simulink model "VTOL_CONTROL_closedloop"  (R2025b)
settings: Solver=VariableStepAuto  StartTime=0.0  StopTime=100  RelTol=1e-3
model workspace (MAT data in the model file):
  M = 1
undefined symbols (not defined in the file): magnitude
libraries: slpidlib x2
settings Model: Creator=Admin  LastModifiedBy=Admin

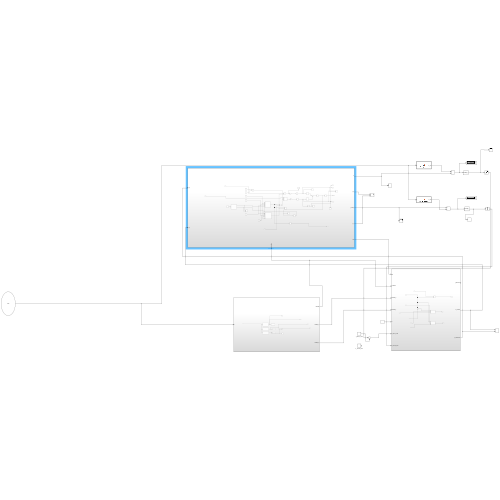
[thumbnail: Simulink's stored preview of the top-level diagram]
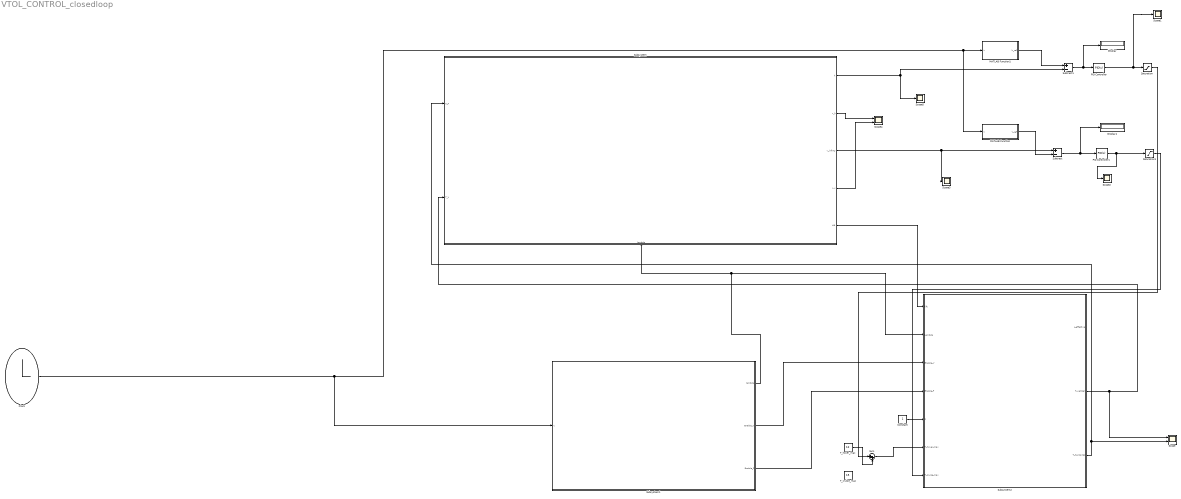
== system VTOL_CONTROL_closedloop ==
  Clock : Clock
      settings: Decimation=100
  Constant : Constant
  Display : Display
  Display1 : Display
  MATLAB Function : MATLAB Function  TreatAsAtomicUnit=on
  MATLAB Function1 : MATLAB Function  TreatAsAtomicUnit=on
  PID Controller : slpidlib/PID Controller  Controller=PID  Form=Parallel  TimeDomain=Continuous-time  UseExternalTs=off  SampleTime=-1  IntegratorMethod=Forward Euler  FilterMethod=Forward Euler  ControllerParametersSource=internal  P=40  I=0  UseKiTs=off  D=25  UseExternalDerivativeSource=off  N=100  UseFilter=on  TunerSelectOption=Transfer Function Based (PID Tuner App)  InitialConditionSource=internal  InitialConditionForIntegrator=0  InitialConditionForFilter=0  DifferentiatorICPrevScaledInput=0  ExternalReset=none  TrackingMode=off  Kt=1  LimitOutput=off  SatLimitsSource=internal  UpperSaturationLimit=inf  LowerSaturationLimit=-inf  LinearizeAsGain=on  AntiWindupMode=none  Kb=1  LimitIntegrator=off  UpperIntegratorSaturationLimit=inf  LowerIntegratorSaturationLimit=-inf  POutMin=[]  POutMax=[]  IOutMin=[]  IOutMax=[]  DOutMin=[]  DOutMax=[]  NOutMin=[]  NOutMax=[]  SumOutMin=[]  SumOutMax=[]  SaturationOutMin=[]  SaturationOutMax=[]  PParamMin=[]  PParamMax=[]  IParamMin=[]  IParamMax=[]  DParamMin=[]  DParamMax=[]  NParamMin=[]  NParamMax=[]  KbParamMin=[]  KbParamMax=[]  KtParamMin=[]  KtParamMax=[]  KbOutMin=[]  KbOutMax=[]  KtOutMin=[]  KtOutMax=[]  IntegratorOutMin=[]  IntegratorOutMax=[]  FilterOutMin=[]  FilterOutMax=[]  SumI1OutMin=[]  SumI1OutMax=[]  SumI2OutMin=[]  SumI2OutMax=[]  SumI3OutMin=[]  SumI3OutMax=[]  SumI4OutMin=[]  SumI4OutMax=[]  SumDOutMin=[]  SumDOutMax=[]  DifferentiatorOutMin=[]  DifferentiatorOutMax=[]  FilterDiffOutCoefMin=[]  FilterDiffOutCoefMax=[]  ReciprocalOutMin=[]  ReciprocalOutMax=[]  SumDenOutMin=[]  SumDenOutMax=[]  SumNumOutMin=[]  SumNumOutMax=[]  DivideOutMin=[]  DivideOutMax=[]  UdiffTsProdOutMin=[]  UdiffTsProdOutMax=[]  NTsProdOutMin=[]  NTsProdOutMax=[]  UintegralTsProdOutMin=[]  UintegralTsProdOutMax=[]  UngainTsProdOutMin=[]  UngainTsProdOutMax=[]  ClampingZeroOutDataTypeStr=Inherit: Inherit via back propagation  ClampingZeroOutMin=[]  ClampingZeroOutMax=[]  FilterDenConstantOutDataTypeStr=Inherit: Inherit via back propagation  FilterDenConstantOutMin=[]  FilterDenConstantOutMax=[]  PCopyOutDataTypeStr=Inherit: Inherit via back propagation  PCopyOutMin=[]  PCopyOutMax=[]  NCopyOutDataTypeStr=Inherit: Inherit via back propagation  NCopyOutMin=[]  NCopyOutMax=[]  IntegratorContinuousStateAttributes=''  IntegratorStateMustResolveToSignalObject=off  IntegratorRTWStateStorageClass=Auto  FilterContinuousStateAttributes=''  FilterStateMustResolveToSignalObject=off  FilterRTWStateStorageClass=Auto  ParallelPVariant=InternalParameters  IdealPVariant=Disabled  IVariant=InternalParameters  DVariant=InternalParameters  IntegratorVariant=Continuous  SatVariant=Disabled  AWVariant=Passthrough  PCopyVariant=Disabled  TRVariant=Disabled  FdbkBlocksVariant=Forward  IdealPFdbkVariant=Disabled  SatFdbkVariant=Disabled  DerivativeFilterVariant=ContFilter  NVariant=InternalParameters  NCopyVariant=Disabled  FilterICVariant=InternalICsFilter  IntegratorICVariant=InternalICs  ExternalResetVariant=Disabled  TRSumVariant=Passthrough  SumFdbkVariant=Disabled  SumVariant=Sum_PID  TsampFilterVariant=InternalTs  TsampNgainVariant=Passthrough  TsampIntegralVariant=Disabled_SignalSpec  ExternalSaturationOutDataTypeStr=Inherit: Same as second input  DerivativeSourceVariant=ErrorSignal  PreIntVariant=InternalPreInt
  PID Controller1 : slpidlib/PID Controller  Controller=PID  Form=Parallel  TimeDomain=Continuous-time  UseExternalTs=off  SampleTime=-1  IntegratorMethod=Forward Euler  FilterMethod=Forward Euler  ControllerParametersSource=internal  P=5  I=0  UseKiTs=off  D=3  UseExternalDerivativeSource=off  N=100  UseFilter=on  TunerSelectOption=Transfer Function Based (PID Tuner App)  InitialConditionSource=internal  InitialConditionForIntegrator=0  InitialConditionForFilter=0  DifferentiatorICPrevScaledInput=0  ExternalReset=none  TrackingMode=off  Kt=1  LimitOutput=off  SatLimitsSource=internal  UpperSaturationLimit=inf  LowerSaturationLimit=-inf  LinearizeAsGain=on  AntiWindupMode=none  Kb=1  LimitIntegrator=off  UpperIntegratorSaturationLimit=inf  LowerIntegratorSaturationLimit=-inf  POutMin=[]  POutMax=[]  IOutMin=[]  IOutMax=[]  DOutMin=[]  DOutMax=[]  NOutMin=[]  NOutMax=[]  SumOutMin=[]  SumOutMax=[]  SaturationOutMin=[]  SaturationOutMax=[]  PParamMin=[]  PParamMax=[]  IParamMin=[]  IParamMax=[]  DParamMin=[]  DParamMax=[]  NParamMin=[]  NParamMax=[]  KbParamMin=[]  KbParamMax=[]  KtParamMin=[]  KtParamMax=[]  KbOutMin=[]  KbOutMax=[]  KtOutMin=[]  KtOutMax=[]  IntegratorOutMin=[]  IntegratorOutMax=[]  FilterOutMin=[]  FilterOutMax=[]  SumI1OutMin=[]  SumI1OutMax=[]  SumI2OutMin=[]  SumI2OutMax=[]  SumI3OutMin=[]  SumI3OutMax=[]  SumI4OutMin=[]  SumI4OutMax=[]  SumDOutMin=[]  SumDOutMax=[]  DifferentiatorOutMin=[]  DifferentiatorOutMax=[]  FilterDiffOutCoefMin=[]  FilterDiffOutCoefMax=[]  ReciprocalOutMin=[]  ReciprocalOutMax=[]  SumDenOutMin=[]  SumDenOutMax=[]  SumNumOutMin=[]  SumNumOutMax=[]  DivideOutMin=[]  DivideOutMax=[]  UdiffTsProdOutMin=[]  UdiffTsProdOutMax=[]  NTsProdOutMin=[]  NTsProdOutMax=[]  UintegralTsProdOutMin=[]  UintegralTsProdOutMax=[]  UngainTsProdOutMin=[]  UngainTsProdOutMax=[]  ClampingZeroOutDataTypeStr=Inherit: Inherit via back propagation  ClampingZeroOutMin=[]  ClampingZeroOutMax=[]  FilterDenConstantOutDataTypeStr=Inherit: Inherit via back propagation  FilterDenConstantOutMin=[]  FilterDenConstantOutMax=[]  PCopyOutDataTypeStr=Inherit: Inherit via back propagation  PCopyOutMin=[]  PCopyOutMax=[]  NCopyOutDataTypeStr=Inherit: Inherit via back propagation  NCopyOutMin=[]  NCopyOutMax=[]  IntegratorContinuousStateAttributes=''  IntegratorStateMustResolveToSignalObject=off  IntegratorRTWStateStorageClass=Auto  FilterContinuousStateAttributes=''  FilterStateMustResolveToSignalObject=off  FilterRTWStateStorageClass=Auto  ParallelPVariant=InternalParameters  IdealPVariant=Disabled  IVariant=InternalParameters  DVariant=InternalParameters  IntegratorVariant=Continuous  SatVariant=Disabled  AWVariant=Passthrough  PCopyVariant=Disabled  TRVariant=Disabled  FdbkBlocksVariant=Forward  IdealPFdbkVariant=Disabled  SatFdbkVariant=Disabled  DerivativeFilterVariant=ContFilter  NVariant=InternalParameters  NCopyVariant=Disabled  FilterICVariant=InternalICsFilter  IntegratorICVariant=InternalICs  ExternalResetVariant=Disabled  TRSumVariant=Passthrough  SumFdbkVariant=Disabled  SumVariant=Sum_PID  TsampFilterVariant=InternalTs  TsampNgainVariant=Passthrough  TsampIntegralVariant=Disabled_SignalSpec  ExternalSaturationOutDataTypeStr=Inherit: Same as second input  DerivativeSourceVariant=ErrorSignal  PreIntVariant=InternalPreInt
  Saturation : Saturate  UpperLimit=12  LowerLimit=0
  Saturation1 : Saturate  UpperLimit=15  LowerLimit=0
  Scope : Scope  NumInputPorts=2
      settings: ActiveDisplayYMinimum=-10.735575752229602  ActiveDisplayYMaximum=32.777554789431129  DataLoggingVariableName=ScopeData3
  Scope{1..3,5} (4 alike) : Scope
      Scope1 settings: ActiveDisplayYMinimum=-82892.5167352317  ActiveDisplayYMaximum=288308.66966188647  DataLoggingVariableName=ScopeData4
      Scope2 settings: ActiveDisplayYMinimum=-3.1458449450480908E+11  ActiveDisplayYMaximum=5.2275837816463568E+11  DataLoggingVariableName=ScopeData5
      Scope3 settings: ActiveDisplayYMinimum=-4.2079891663951721E+10  ActiveDisplayYMaximum=1.3406215699659059E+11  DataLoggingVariableName=ScopeData6
      Scope5 settings: ActiveDisplayYMinimum=-3.5700117220620872E+16  ActiveDisplayYMaximum=3.4956584287541544E+16  DataLoggingVariableName=ScopeData8
  Scope4 : Scope  NumInputPorts=2
      settings: ActiveDisplayYMinimum=-8.1957611797470367E+10  ActiveDisplayYMaximum=4.5711328699465958E+10  DataLoggingVariableName=ScopeData7
  Subsystem : Subsystem
      settings: PortSchema="{\"entries\":[{\"content\":{\"sides\":[{\"content\":{\"connectorIds\":[\"In1\",\"In2\"]},\"type\":\"ConnectorPlacement.EquallySpacedRectSide\",\"uuid\":\"717a2cf3-1c0a-44a3-a2ba-538b072e1925\"},{\"content\":{\"connectorIds\":[\"Out1\",\"Out2\",\"Out3\",\"Out4\",\"Out5\"],\"side\":\"RIGHT\"},\"type\":\"ConnectorPlacement.EquallySpacedRectSide\",\"uuid\":\"4d25b5c0-f552-4ea0-9a18-e627fc8b4c8d\"},{\"content\":{\"side\":\"TOP\"},\"type\":\"ConnectorPlacement.EquallySpacedRectSide\",\"uuid\":\"5e6d914d-af3e-475b-a39c-cb9752cea2cc\"},{\"content\":{\"connectorIds\":[\"In3\"],\"side\":\"BOTTOM\"},\"type\":\"ConnectorPlacement.EquallySpacedRectSide\",\"uuid\":\"37b414cc-fcce-4794-8705-d953038efecc\"}]},\"type\":\"ConnectorPlacement.EquallySpacedConnector\",\"uuid\":\"6ac88909-4469-4441-8145-ec1acf4a18cc\"}],\"packageUris\":[\"http://schema.mathworks.com/mf0/Connector/R2020b\"],\"version\":\"1.0\"}"
  Subsystem1 : Subsystem
  Subsystem2 : Subsystem
  Subtract : Sum  Inputs=+-
  Subtract1 : Sum  Inputs=+-
  Sum : Sum  Inputs=|++
  T_cruise_max : Constant  Value=15
  T_hover_max : Constant  Value=12
  wires:
  Subtract/1 -> Display1/1, PID Controller1/1
  PID Controller/1 -> Saturation/1, Scope1/1
  PID Controller1/1 -> Scope2/1, Saturation1/1
  MATLAB Function1/1(h_ref) -> Subtract1/1
  Subtract1/1 -> Display/1, PID Controller/1
  MATLAB Function/1(V_ref) -> Subtract/2
  Clock/1 -> MATLAB Function/1(t), MATLAB Function1/1(t), Subsystem1/1(t)
  Subsystem1/1(lambda) -> Subsystem2/2(Lambda), Subsystem/3(lambda)
  Subsystem/3(v_infinty) -> Scope3/1, Subtract/1
  Subsystem/1(h) -> Scope5/1, Subtract1/2
  Subsystem2/2(T_vertical) -> Scope/1, Subsystem/2(T_V)
  Subsystem1/2(Enable_V) -> Subsystem2/3(Enable_V)
  Subsystem/5(Lift) -> Subsystem2/1(lift)
  Subsystem2/3(T_horizontal) -> Scope/2, Subsystem/1(T_F)
  Subsystem1/3(Enable_F) -> Subsystem2/4(Enable_F)
  Constant/1 -> Subsystem2/5(1)
  Saturation1/1 -> Subsystem2/7(T_cruise_max)
  T_hover_max/1 -> Sum/2
  Saturation/1 -> Sum/1
  Sum/1 -> Subsystem2/6(T_hover_max)
  Subsystem/2(v_h) -> Scope4/1
  Subsystem/4(v_v) -> Scope4/2

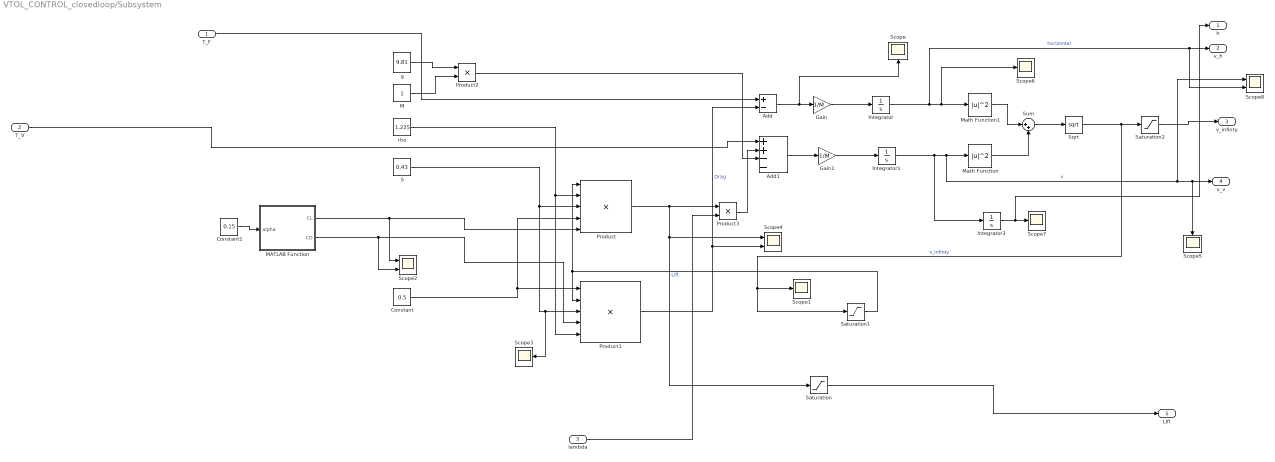
== system VTOL_CONTROL_closedloop/Subsystem ==
  T_F : Inport
  T_V : Inport  Port=2
  lambda : Inport  Port=3
  Add : Sum  Inputs=+-
  Add1 : Sum  Inputs=++--
  Constant : Constant  Value=0.5
  Constant1 : Constant  Value=0.15
  Gain : Gain  Gain=1/M
  Gain1 : Gain  Gain=1/M
  Integrator : Integrator
  Integrator1 : Integrator
  Integrator3 : Integrator
  M : Constant
  MATLAB Function : MATLAB Function  TreatAsAtomicUnit=on
  Math Function : Math  Operator=magnitude^2
  Math Function1 : Math  Operator=magnitude^2
  Product : Product  Inputs=5
  Product1 : Product  Inputs=5
  Product2 : Product
  Product3 : Product
  S : Constant  Value=0.43
  Saturation : Saturate  UpperLimit=10  LowerLimit=0
  Saturation1 : Saturate  UpperLimit=5  LowerLimit=0
  Saturation2 : Saturate  UpperLimit=5  LowerLimit=0
  Scope{,1,3,5..7} (6 alike) : Scope
      Scope settings: ActiveDisplayYMinimum=-8.88786252335554  ActiveDisplayYMaximum=13.902879664144468  DataLoggingVariableName=ScopeData9
      Scope1 settings: ActiveDisplayYMinimum=-1.5960606995519469E+9  ActiveDisplayYMaximum=1.7060905559873872E+9  DataLoggingVariableName=ScopeData10
      Scope3 settings: ActiveDisplayYMinimum=0.34836157841071735  ActiveDisplayYMaximum=0.52112909811701269  DataLoggingVariableName=ScopeData12
      Scope5 settings: ActiveDisplayYMinimum=-532.97175373907817  ActiveDisplayYMaximum=160.0455368180661  DataLoggingVariableName=ScopeData14
      Scope6 settings: ActiveDisplayYMinimum=-6.5098067230662071  ActiveDisplayYMaximum=2.0724636667868079  DataLoggingVariableName=ScopeData15
      Scope7 settings: ActiveDisplayYMinimum=-25989.976839496954  ActiveDisplayYMaximum=10776.010068154665  DataLoggingVariableName=ScopeData16
  Scope2 : Scope  NumInputPorts=2
      settings: ActiveDisplayYMinimum=-1  ActiveDisplayYMaximum=1  DataLoggingVariableName=ScopeData11
  Scope4 : Scope  NumInputPorts=2
      settings: ActiveDisplayYMinimum=-1  ActiveDisplayYMaximum=1  DataLoggingVariableName=ScopeData13
  Scope8 : Scope  NumInputPorts=2
      settings: ActiveDisplayYMinimum=-465.71565679884253  ActiveDisplayYMaximum=132.93873521683119  DataLoggingVariableName=ScopeData17
  Sqrt : Sqrt
  Sum : Sum  Inputs=|++
  g : Constant  Value=9.81
  rho : Constant  Value=1.225
  h : Outport
  v_h : Outport  Port=2
  v_infinty : Outport  Port=3
  v_v : Outport  Port=4
  Lift : Outport  Port=5
  wires:
  Integrator/1 -> Scope8/2, v_h/1, Scope6/1, Math Function1/1  "horizontal"
  Gain/1 -> Integrator/1
  Add/1 -> Scope/1, Gain/1
  rho/1 -> Product1/5, Product/2
  Add1/1 -> Gain1/1
  S/1 -> Scope3/1, Product1/3, Product/3
  Constant/1 -> Product/4, Product1/1
  Product1/1 -> Scope4/2, Add/2  "Drag"
  Sqrt/1 -> Scope1/1, Saturation1/1, Saturation2/1  "v_infinty"
  MATLAB Function/2(CD) -> Scope2/2, Product1/4
  Integrator1/1 -> Integrator3/1, v_v/1, Scope5/1, Scope8/1, Math Function/1  "v"
  Product/1 -> Saturation/1, Scope4/1, Product3/1  "Lift"
  g/1 -> Product2/1
  MATLAB Function/1(CL) -> Scope2/1, Product/5
  Product2/1 -> Add1/3
  Math Function1/1 -> Sum/1
  Math Function/1 -> Sum/2
  M/1 -> Product2/2
  Gain1/1 -> Integrator1/1
  Sum/1 -> Sqrt/1
  T_F/1 -> Add/1
  T_V/1 -> Add1/1
  Product3/1 -> Add1/2
  lambda/1 -> Product3/2
  Saturation/1 -> Lift/1
  Constant1/1 -> MATLAB Function/1(alpha)
  Saturation1/1 -> Product/1, Product1/2
  Saturation2/1 -> v_infinty/1
  Integrator3/1 -> h/1, Scope7/1

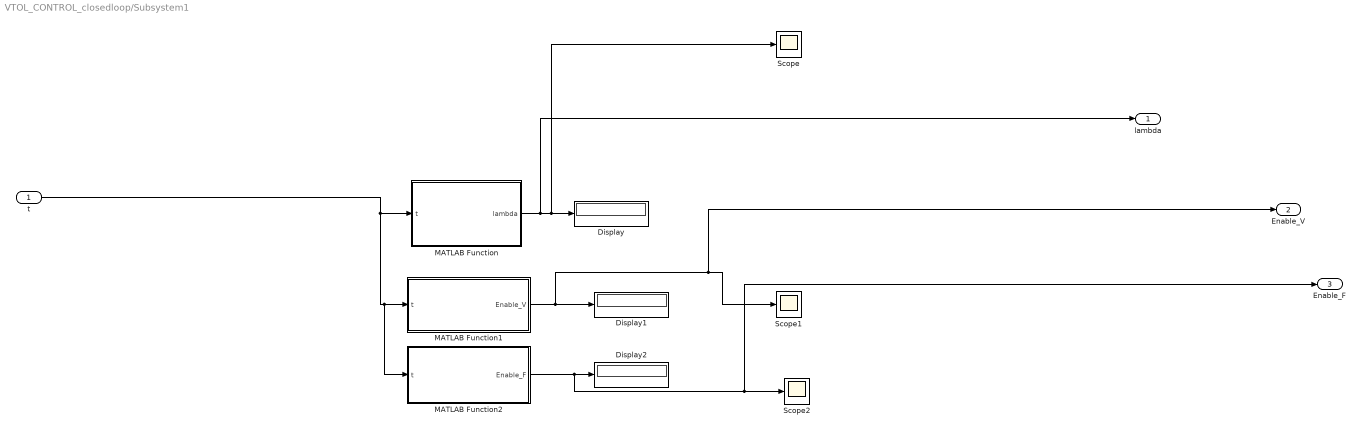
== system VTOL_CONTROL_closedloop/Subsystem1 ==
  t : Inport
  Display : Display
  Display1 : Display
  Display2 : Display
  MATLAB Function : MATLAB Function  TreatAsAtomicUnit=on
  MATLAB Function1 : MATLAB Function  TreatAsAtomicUnit=on
  MATLAB Function2 : MATLAB Function  TreatAsAtomicUnit=on
  Scope : Scope
      settings: ActiveDisplayYMinimum=-0.32672444487235941  ActiveDisplayYMaximum=1.3483951059088912
  Scope1 : Scope
      settings: ActiveDisplayYMinimum=-0.35557693733498685  ActiveDisplayYMaximum=1.5835833326381588
  Scope2 : Scope
      settings: ActiveDisplayYMinimum=-1.979172228109352  ActiveDisplayYMaximum=3.6933771392759018  DataLoggingVariableName=ScopeData2
  lambda : Outport
  Enable_V : Outport  Port=2
  Enable_F : Outport  Port=3
  wires:
  MATLAB Function2/1(Enable_F) -> Enable_F/1, Scope2/1, Display2/1
  MATLAB Function/1(lambda) -> lambda/1, Scope/1, Display/1
  t/1 -> MATLAB Function2/1(t), MATLAB Function1/1(t), MATLAB Function/1(t)
  MATLAB Function1/1(Enable_V) -> Enable_V/1, Scope1/1, Display1/1

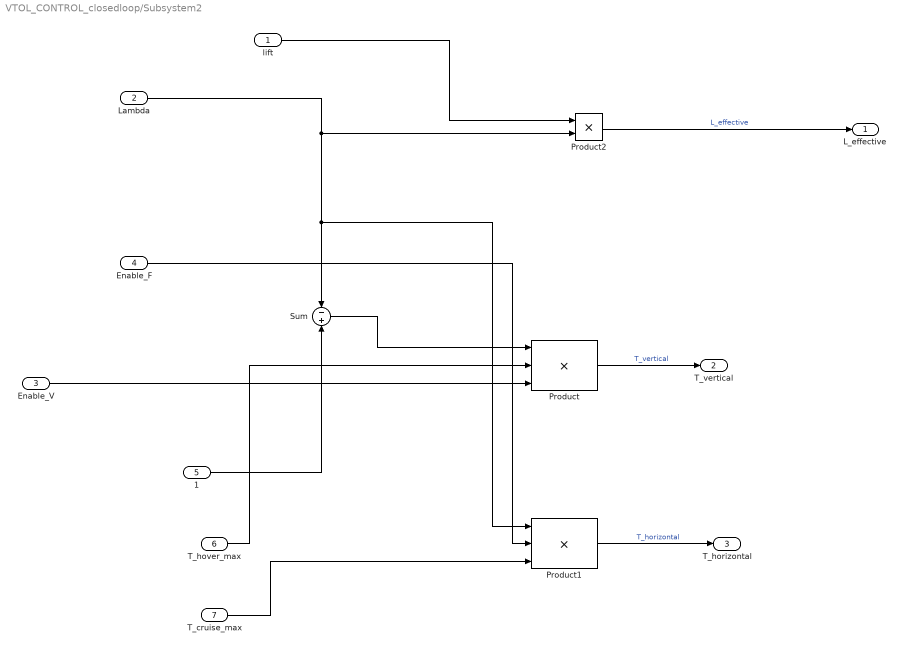
== system VTOL_CONTROL_closedloop/Subsystem2 ==
  lift : Inport
  Lambda : Inport  Port=2
  Enable_V : Inport  Port=3
  Enable_F : Inport  Port=4
  1 : Inport  Port=5
  T_hover_max : Inport  Port=6
  T_cruise_max : Inport  Port=7
  Product : Product  Inputs=3
  Product1 : Product  Inputs=3
  Product2 : Product
  Sum : Sum  Inputs=-+
  L_effective : Outport
  T_vertical : Outport  Port=2
  T_horizontal : Outport  Port=3
  wires:
  T_hover_max/1 -> Product/2
  Sum/1 -> Product/1
  Lambda/1 -> Product2/2, Product1/1, Sum/1
  Enable_F/1 -> Product1/2
  Product/1 -> T_vertical/1  "T_vertical"
  Product1/1 -> T_horizontal/1  "T_horizontal"
  lift/1 -> Product2/1
  Enable_V/1 -> Product/3
  1/1 -> Sum/2
  Product2/1 -> L_effective/1  "L_effective"
  T_cruise_max/1 -> Product1/3

== matlab function VTOL_CONTROL_closedloop/Subsystem1/MATLAB Function ==
  data: lambda output; t input
function lambda = blend_factor(t)

if t < 10
    lambda = 0;

elseif t < 30
    a = (t - 10)/20;      % normalized time 0→1
    lambda = a^2;        % parabolic ramp up

elseif t < 65
    lambda = 1;

else
    a = (t - 65)/35;     % normalized time 0→1
    lambda = 1 - a^2;   % parabolic ramp down
end

== matlab function VTOL_CONTROL_closedloop/Subsystem1/MATLAB Function2 ==
  data: t input; Enable_F output
function Enable_F = enable_forward(t)

% Forward thrust enable logic

if t > 10 && t < 55
    Enable_F = true;     % Transition + Cruise
else
    Enable_F = false;    % Hover, Glide, Back transition
end

== matlab function VTOL_CONTROL_closedloop/MATLAB Function ==
  data: t input; V_ref output
function V_ref = airspeed_reference(t)

V_cruise = 20;   % m/s (choose realistic value)

if t < 10
    V_ref = 0;   % Hover

elseif t < 30
    % Smooth ramp-up (10–30 s)
    tau = (t - 10)/20;
    tau = min(max(tau,0),1);
    V_ref = V_cruise * (3*tau^2 - 2*tau^3);

elseif t < 65
    V_ref = V_cruise;   % Cruise + Glide

else
    % Back transition (65–85 s)
    tau = (t - 65)/20;
    tau = min(max(tau,0),1);
    V_ref = V_cruise * (1 - (3*tau^2 - 2*tau^3));
end

end

== matlab function VTOL_CONTROL_closedloop/MATLAB Function1 ==
  data: t input; h_ref output
function h_ref = altitude_reference(t)

h_hover  = 100;   % m
h_cruise = 95;    % m (slight drop after transition)
h_glide  = 70;    % m (target glide altitude)

if t < 10
    h_ref = h_hover;   % Hover

elseif t < 30
    % Smooth drop (transition)
    tau = (t - 10)/20;
    tau = min(max(tau,0),1);
    h_ref = h_hover - (h_hover - h_cruise)*(3*tau^2 - 2*tau^3);

elseif t < 55
    h_ref = h_cruise;  % Cruise

elseif t < 65
    % Glide descent
    tau = (t - 55)/10;
    tau = min(max(tau,0),1);
    h_ref = h_cruise - (h_cruise - h_glide)*tau;

else
    % Back transition climb
    tau = (t - 65)/20;
    tau = min(max(tau,0),1);
    h_ref = h_glide + (h_hover - h_glide)*(3*tau^2 - 2*tau^3);
end

end

== matlab function VTOL_CONTROL_closedloop/Subsystem/MATLAB Function ==
  data: alpha input; CL output; CD output
function [CL, CD] = aero_coeff(alpha)

% -------------------------------------------------
% Aerodynamic coefficients (from literature / CFD)
% Reference: Yuksek et al., 2016
% -------------------------------------------------

% ---- Parameters ----
CL0      = 0.124;        % Lift coefficient at alpha = 0 (3D CFD)
CL_alpha = 4.2;          % Lift slope (per rad)

CD0      = 0.032;        % Zero-lift drag coefficient (3D CFD)
k        = 0.08;         % Induced drag factor

% ---- Angle of attack limits (safety) ----
alpha = max(min(alpha, deg2rad(15)), deg2rad(-10));

% ---- Lift coefficient ----
CL = CL0 + CL_alpha * alpha;

% ---- Drag coefficient (parabolic model) ----
CD = CD0 + k * CL^2;

end

== matlab function VTOL_CONTROL_closedloop/Subsystem1/MATLAB Function1 ==
  data: t input; Enable_V output
function Enable_V = enable_vertical(t)

% Vertical thrust enable logic

if t < 55
    Enable_V = true;     % Hover + Transition + Cruise entry
elseif t >= 65
    Enable_V = true;     % Back transition
else
    Enable_V = false;    % Glide phase (55–65 s)
end
